simulink model "num2"  (R2018b)
settings: Solver=FixedStepAuto  StartTime=0.0  StopTime=10.0  FixedStep=0.02  RelTol=1e-3
settings Model: Creator=reema  LastModifiedBy=reema

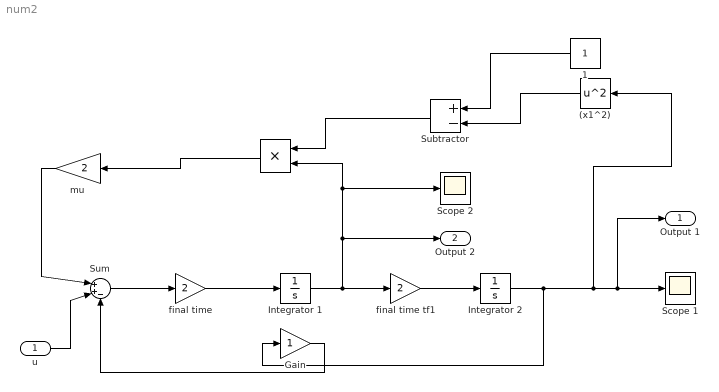
== system num2 ==
  u : Inport
  " " : Product
  (x1^2) : Math  Operator=square  SaturateOnIntegerOverflow=on
  1 : Constant
  Gain : Gain
  Integrator 1 : Integrator
  Integrator 2 : Integrator
  Scope 1 : Scope
  Scope 2 : Scope
  Subtractor : Sum  Inputs=+-
  Sum : Sum  Inputs=|++-
  final time : Gain  Gain=2
  final time tf1 : Gain  Gain=2
  mu : Gain  Gain=2
  Output 1 : Outport
  Output 2 : Outport  Port=2
  wires:
  1/1 -> Subtractor/1
  final time tf1/1 -> Integrator 2/1
  Integrator 2/1 -> (x1^2)/1, Output 1/1, Scope 1/1, Gain/1
  (x1^2)/1 -> Subtractor/2
  Subtractor/1 -> " "/1
  Sum/1 -> final time/1
  u/1 -> Sum/2
  Integrator 1/1 -> final time tf1/1, " "/2, Scope 2/1, Output 2/1
  " "/1 -> mu/1
  final time/1 -> Integrator 1/1
  mu/1 -> Sum/1
  Gain/1 -> Sum/3
